simulink model "pv_mppt_inverter"  (R2014a)
settings: Solver=ode23tb  StartTime=0.0  StopTime=1  RelTol=1e-3
PreLoadFcn:
  | load('DCDCBuck_Variants');
  | load('DCACInverter_Variants');
  | load('MPPT_Variants');
  | BuckMode = 1;
  | InvMode = 1;
  | MPPTMode = 1;
  | Ts = 1e-6;
  | G = 1000;
  | PVCellIsc = 7;
  | PVCellVoc = 0.64;
  | PVCellRs = 0.001;
  | tau = 1e-4;
undefined symbols (not defined in the file or in its folder): D1, Delta, dfilt, sigbuilder_block
libraries: powerlib x48, powerlib_meascontrol x8, dsparch4 x3, simulink_extras x3, simulink x2
settings Model: Creator=cosorio  LastModifiedBy=cosorio
settings DataIOCC: LimitDataPoints=off  SignalLoggingSaveFormat=ModelDataLogs  SaveOutput=off  SignalLogging=off  DSMLogging=off  SaveTime=off  OutputTimes=[0]
settings OptimizationCC: ExpressionDepthLimit=2147483647
settings DebuggingCC: UnderspecifiedInitializationDetection=Classic  FcnCallInpInsideContextMsg=UseLocalSettings  StateNameClashWarn=warning
settings GRTTargetCC: CombineOutputUpdateFcns=off  GRTInterface=on

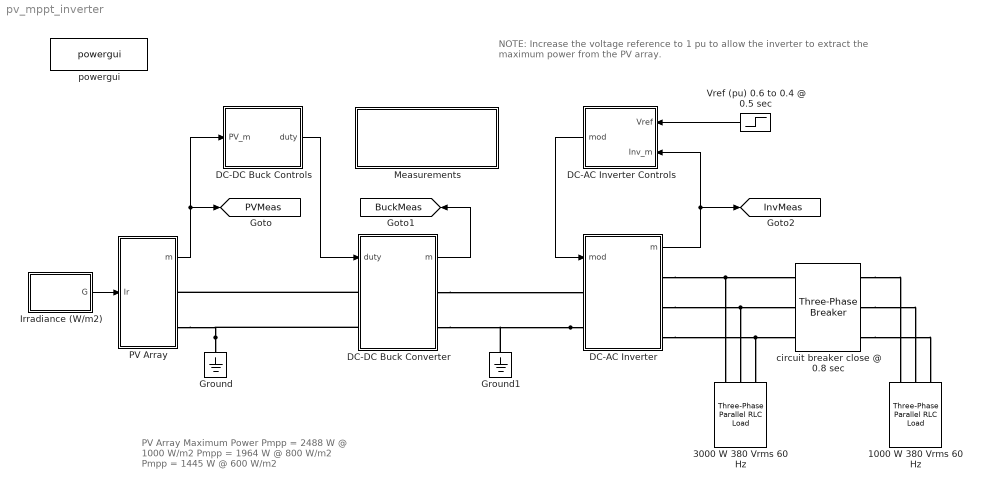
== system pv_mppt_inverter ==
  note: PV Array Maximum Power
      | Pmpp = 2488 W @ 1000 W/m2
      | Pmpp = 1964 W @ 800 W/m2
      | Pmpp = 1445 W @ 600 W/m2
  note: NOTE: Increase the voltage reference to 1 pu to allow the
      | inverter to extract the maximum power from the PV array.
  1000 W 380 Vrms 60 Hz : powerlib/Elements/Three-Phase Parallel RLC Load  LConnTagsString=A|B|C  Configuration=Y (grounded)  NominalVoltage=380  NominalFrequency=60  ActivePower=1000  InductivePower=0  CapacitivePower=0  Measurements=None  LoadType=constant Z
  3000 W 380 Vrms 60 Hz : powerlib/Elements/Three-Phase Parallel RLC Load  LConnTagsString=A|B|C  Configuration=Y (grounded)  NominalVoltage=380  NominalFrequency=60  ActivePower=3000  InductivePower=0  CapacitivePower=0  Measurements=None  LoadType=constant Z
  DC-AC Inverter : Subsystem  Variant=on
  DC-AC Inverter Controls : Subsystem  TreatAsAtomicUnit=on  SystemSampleTime=1e-4
  DC-DC Buck Controls : Subsystem  TreatAsAtomicUnit=on  SystemSampleTime=1e-4
  DC-DC Buck Converter : Subsystem  Variant=on
  Ground : powerlib/Elements/Ground  LConnTagsString=a
  Ground1 : powerlib/Elements/Ground  LConnTagsString=a
  Irradiance (W/m2) : Subsystem  Tag=STV Subsys  LoadFcn=sigbuilder_block('load');  StartFcn=sigbuilder_block('start');  StopFcn=sigbuilder_block('stop');  ClipboardFcn=sigbuilder_block('clipboard');  mask(Sigbuilder block){}
      mask help: Sigbuilder GUI
      mask init:
      | if ~strcmp(get_param(bdroot(gcbh),'SimulationStatus'),'stopped') tuvar = sigbuilder_block('maskInit'); end
      settings: CopyFcn=sigbuilder_block('copy');  DeleteFcn=sigbuilder_block('delete');  ModelCloseFcn=sigbuilder_block('modelClose');  PreSaveFcn=sigbuilder_block('preSave');  PauseFcn=sigbuilder_block('pause')  ContinueFcn=sigbuilder_block('continue')  NameChangeFcn=sigbuilder_block('namechange');  OpenFcn=sigbuilder_block('open',[124.138 6.82759 550.552 382.345 ]);  CloseFcn=sigbuilder_block('close');
      mask Display: plot(0,0,100,100,[10,10,40,40,10],[80,20,20,80,80],[40,10],[50,50], [40,27,10],[65,72,56],[40,25,25,10],[28,28,43,43]);
  Measurements : Subsystem
      mask Display: disp('System\nMeasurements');
  PV Array : Subsystem
  Vref (pu) 0.6 to 0.4 @ 0.5 sec : Step  Time=0.5  Before=0.6  After=0.4  SampleTime=1e-4
  circuit breaker close @ 0.8 sec : powerlib/Elements/Three-Phase Breaker  InitialState=open  SwitchA=on  SwitchB=on  SwitchC=on  SwitchTimes=[0.8]  External=off  BreakerResistance=0.001  SnubberResistance=1e6  SnubberCapacitance=inf  Measurements=None
  powergui : powerlib/powergui  Priority=1  SimulationMode=Continuous  SolverType=Tustin  SampleTime=Ts  frequency=60  SPID=off  DisableSnubberDevices=off  DisableRonSwitches=off  DisableVfSwitches=off  SwTol=0  Interpol=off  DisplayEquations=off  Ts=0  methode=off  frequencyindice=0  Pbase=100e6  ErrMax=1e-4  Iterations=50  UnitsV=kV  UnitsW=MW  FunctionMessages=off  echomessages=off  HookPort=off  EnableUseOfTLC=off  x0status=blocks  RestoreLinks=warning  ResistiveCurrentMeasurement=off  Frange=[0:2:500]  Ylog=off  Xlog=on  ShowGrid=off  save=off  variable=ZData  structure=InverterData  ZoomFFT=off  StartTime=0.1  cycles=3  DisplayStyle=1  fundamental=60  FreqAxis=on  MaxFrequency=24000  frequencyindicesteady=1  RmsSteady=1  display=off
  tag scope: BuckMeas=global, InvMeas=global, PVMeas=global
  wires:
  Irradiance (W/m2)/1(G) -> PV Array/1(Ir)
  DC-DC Buck Controls/1(duty) -> DC-DC Buck Converter/1(duty)
  PV Array/1(m) -> DC-DC Buck Controls/1(PV_m), [PVMeas]
  DC-DC Buck Converter/1(m) -> [BuckMeas]
  DC-AC Inverter/1(m) -> DC-AC Inverter Controls/2(Inv_m), [InvMeas]
  DC-AC Inverter Controls/1(mod) -> DC-AC Inverter/1(mod)
  Vref (pu) 0.6 to 0.4 @ 0.5 sec/1 -> DC-AC Inverter Controls/1(Vref)
  connections:
  Ground/LConn1 -- DC-DC Buck Converter/LConn2 -- PV Array/RConn2
  DC-DC Buck Converter/LConn1 -- PV Array/RConn1
  DC-DC Buck Converter/RConn1 -- DC-AC Inverter/LConn1
  DC-AC Inverter/LConn2 -- DC-DC Buck Converter/RConn2 -- Ground1/LConn1
  DC-AC Inverter/RConn1 -- circuit breaker close @ 0.8 sec/LConn1 -- 3000 W 380 Vrms 60 Hz/LConn1
  DC-AC Inverter/RConn2 -- 3000 W 380 Vrms 60 Hz/LConn2 -- circuit breaker close @ 0.8 sec/LConn2
  DC-AC Inverter/RConn3 -- circuit breaker close @ 0.8 sec/LConn3 -- 3000 W 380 Vrms 60 Hz/LConn3
  circuit breaker close @ 0.8 sec/RConn3 -- 1000 W 380 Vrms 60 Hz/LConn3
  circuit breaker close @ 0.8 sec/RConn2 -- 1000 W 380 Vrms 60 Hz/LConn2
  circuit breaker close @ 0.8 sec/RConn1 -- 1000 W 380 Vrms 60 Hz/LConn1

== system pv_mppt_inverter/DC-AC Inverter ==
  mod : Inport
  AVG Voltage : Subsystem  VariantControl=DCACInverterAVG
  Detailed : Subsystem  VariantControl=DCACInverterDET
  in + : PMIOPort  Port=1  Side=Left
  in -- : PMIOPort  Port=2  Side=Left
  A : PMIOPort  Port=3  Side=Right
  B : PMIOPort  Port=4  Side=Right
  C : PMIOPort  Port=5  Side=Right
  m : Outport

== system pv_mppt_inverter/DC-AC Inverter Controls ==
  note: NOTE: Regulating the inverter to a desired setpoint voltage for
      | a fixed load will limit the current flowing through the inverter.
      | As can be seen from the simulation, this results in the PV array
      | NOT necessarily operating at peak efficiency.
  Vref : Inport  SampleTime=1e-4
  Inv_m : Inport  Port=2  SampleTime=1e-4
  Bus Selector3 : BusSelector  OutputSignals=VabcInv
  Voltage Regulator : Subsystem
  mod : Outport
  wires:
  Bus Selector3/1 -> Voltage Regulator/2(Vabc (pu))  "<VabcInv>"
  Inv_m/1 -> Bus Selector3/1
  Vref/1 -> Voltage Regulator/1(Vd_ref (pu))
  Voltage Regulator/1(Vabc_inv) -> mod/1

== system pv_mppt_inverter/DC-DC Buck Controls ==
  PV_m : Inport  SampleTime=1e-4
  Bus Selector : BusSelector  OutputSignals=PVVocREF (V),PVVoltage (V),PVCurrent (A)
  MPPT Algorithm : ModelReference  ModelNameDialog=FractionalOCVoltage.slx  Variant=on  ModelReferenceVersion=1.167  CopyOfModelName=FractionalOCVoltage.slx  DefaultDataLogging=on
  Signal Conditioning : Subsystem
  duty : Outport
  wires:
  PV_m/1 -> Bus Selector/1
  Bus Selector/2 -> Signal Conditioning/2(In2)  "<PVVoltage (V)>"
  Bus Selector/1 -> Signal Conditioning/1(In1)  "<PVVocREF (V)>"
  MPPT Algorithm/1 -> duty/1
  Signal Conditioning/1(Out1) -> MPPT Algorithm/1
  Signal Conditioning/2(Out2) -> MPPT Algorithm/2
  Bus Selector/3 -> Signal Conditioning/3(In3)  "<PVCurrent (A)>"
  Signal Conditioning/3(Out3) -> MPPT Algorithm/3

== system pv_mppt_inverter/DC-DC Buck Converter ==
  duty : Inport
  AVG Voltage : Subsystem  VariantControl=DCDCBuckAVG
  Detailed : Subsystem  VariantControl=DCDCBuckDET
  Low Level : Subsystem  VariantControl=DCDCBuckLOW
  in + : PMIOPort  Port=1  Side=Left
  in -- : PMIOPort  Port=2  Side=Left
  out + : PMIOPort  Port=3  Side=Right
  out -- : PMIOPort  Port=4  Side=Right
  m : Outport

== system pv_mppt_inverter/Irradiance (W//m2) ==
  Demux : Demux  Tag=STV Demux  Outputs=1
  FromWs : FromWorkspace  Tag=STV FromWs  VariableName=tuvar  SampleTime=0
      SigBuilderData=|
      | common.afterFinalStr = 'Extrapolate'
      | common.sampleTime = '0'
      | dataSet(1).timeRange = [0 1]
      | dataSet(1).name = 'Constant Irradiance'
      | dataSet(2).timeRange = [0 1]
      | dataSet(2).name = 'Step Irradiance'
      | dataSet(3).timeRange = [0 1]
      | dataSet(3).name = 'Trapezoidal Irradiance'
      | sbobj.Groups(1).Name = 'Constant Irradiance'
      | sbobj.Groups(1).Signals.Name = 'G'
      | sbobj.Groups(1).Signals.XData = [0 1]
      | sbobj.Groups(1).Signals.YData = [800 800]
      | sbobj.Groups(1).TimeRange = [0 1]
      | sbobj.Groups(2).Name = 'Step Irradiance'
      | sbobj.Groups(2).Signals.Name = 'G'
      | sbobj.Groups(2).Signals.XData = [0 0.5 0.5 1]
      | sbobj.Groups(2).Signals.YData = [600 600 1000 1000]
      | sbobj.Groups(2).TimeRange = [0 1]
      | sbobj.Groups(3).Name = 'Trapezoidal Irradiance'
      | sbobj.Groups(3).Signals.Name = 'G'
      | sbobj.Groups(3).Signals.XData = [0 0.2 0.3 0.5 0.7 0.9 1]
      | sbobj.Groups(3).Signals.YData = [800 800 600 600 1000 1000 800]
      | sbobj.Groups(3).TimeRange = [0 1]
  G : Outport  Tag=STV Outport
  wires:
  Demux/1 -> G/1
  FromWs/1 -> Demux/1

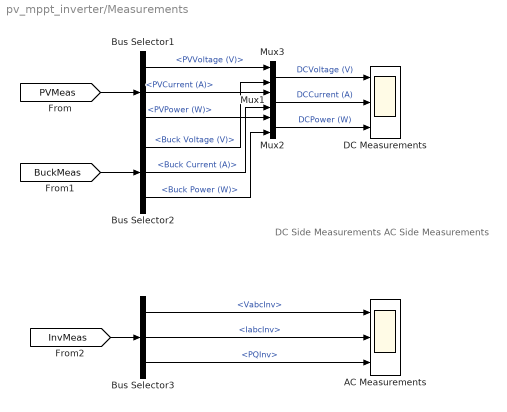
== system pv_mppt_inverter/Measurements ==
  note: DC Side Measurements
      |
      |
      |
      |
      |
      |
      |
      |
      |
      |
      | AC Side Measurements
  AC Measurements : Scope  NumInputPorts=3
      settings: YMin=-2~-1~-0.5  YMax=2~1~1  SaveName=InverterData
  Bus Selector1 : BusSelector  OutputSignals=PVVoltage (V),PVCurrent (A),PVPower (W)
  Bus Selector2 : BusSelector  OutputSignals=Buck Voltage (V),Buck Current (A),Buck Power (W)
  Bus Selector3 : BusSelector  OutputSignals=VabcInv,IabcInv,PQInv
  DC Measurements : Scope  NumInputPorts=3
      settings: YMin=0~0~0  YMax=250~40~3000  SaveName=PVArrayData
  Mux1 : Mux  Inputs=2
  Mux2 : Mux  Inputs=2
  Mux3 : Mux  Inputs=2
  wires:
  Bus Selector1/1 -> Mux3/1  "<PVVoltage (V)>"
  Bus Selector1/2 -> Mux1/1  "<PVCurrent (A)>"
  Bus Selector1/3 -> Mux2/1  "<PVPower (W)>"
  Bus Selector2/1 -> Mux3/2  "<Buck Voltage (V)>"
  Bus Selector2/2 -> Mux1/2  "<Buck Current (A)>"
  Bus Selector2/3 -> Mux2/2  "<Buck Power (W)>"
  Mux3/1 -> DC Measurements/1  "DCVoltage (V)"
  Mux1/1 -> DC Measurements/2  "DCCurrent (A)"
  Mux2/1 -> DC Measurements/3  "DCPower (W)"
  [PVMeas] -> Bus Selector1/1
  [BuckMeas] -> Bus Selector2/1
  [InvMeas] -> Bus Selector3/1
  Bus Selector3/1 -> AC Measurements/1  "<VabcInv>"
  Bus Selector3/2 -> AC Measurements/2  "<IabcInv>"
  Bus Selector3/3 -> AC Measurements/3  "<PQInv>"

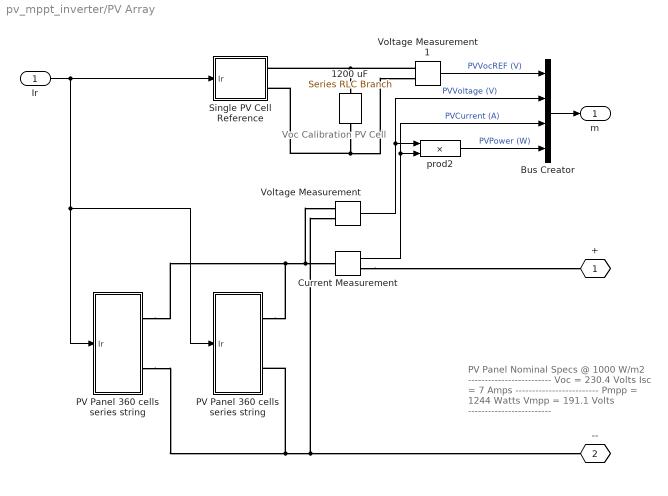
== system pv_mppt_inverter/PV Array ==
  note: Voc Calibration PV Cell
  note: PV Panel
      | Nominal Specs @ 1000 W/m2
      | -------------------------
      | Voc = 230.4 Volts
      | Isc = 7 Amps
      | -------------------------
      | Pmpp = 1244 Watts
      | Vmpp = 191.1 Volts
      | -------------------------
  Ir : Inport
  1200 uF : powerlib/Elements/Series RLC Branch  LConnTagsString=__new0  RConnTagsString=__new0  BranchType=C  Resistance=0.05  Inductance=1e-3  SetiL0=off  InitialCurrent=0  Capacitance=1200e-6  Setx0=on  InitialVoltage=PVCellVoc  Measurements=None
  Bus Creator : BusCreator
  Current Measurement : powerlib/Measurements/Current Measurement  PhasorSimulation=off  OutputType=Complex  PSBequivalent=0
  PV Panel 360 cells series string : Subsystem  mask(Solar Cell){Isc=PVCellIsc, Voc=PVCellVoc*360, Ir0=1000, N=1.5*360, Rs=PVCellRs*360, Rp=1000*360, tau=tau}
      mask prompts: Isc "Short-circuit current, Isc (A):"; Voc "Open-circuit voltage, Voc (V):"; Ir0 "Irradiance used for measurements, Ir0 (W/m2):"; N "Quality factor, N:"; Rs "Series resistance, Rs (ohms):"; Rp "Parallel resistance, Rp (ohms):"; tau "Time constant (sec):"
      mask help:
      | Simulink implementation of an idividual solar cell. The cell is modelled as a parallel combination of a current source, an exponential diode and an internal resistance Rp, connected in series with a resistance Rs.
      | The cell output current is given by:
      |
      | Ipv = Iph - Is * (exp((V + I*Rs)/(N*Vt)) - 1) - (V + I*Rs)/Rp
      |
      | Where Iph is the solar generated current, Is is the diode saturation current, Vt is the thermal voltage, N is the diode quality factor (emission coefficient).
      |
      | A first order transfer function is used to break the algebraic loop. The time constant of this transfer function should be adjusted such that it will not significantly affect your model dynamics.
      mask init:
      | %% Cell thermal voltage calculation
      | T = 25 + 273;   % Device operating temperature (oC)
      | k = 1.3806e-23; % Boltzman constant (J/oK)
      | q = 1.602e-19;  % Elementary charge on an electron (oC)
      | Vt = k*T/q;     % Thermal voltage
      | 
      | %% Diode saturation current calculation
      | Is = Isc/(exp(Voc/(N*Vt))-1);
  "PV Panel 360 cells series string " : Subsystem  mask(Solar Cell){Isc=PVCellIsc, Voc=PVCellVoc*360, Ir0=1000, N=1.5*360, Rs=PVCellRs*360, Rp=1000*360, tau=tau}
      mask prompts: Isc "Short-circuit current, Isc (A):"; Voc "Open-circuit voltage, Voc (V):"; Ir0 "Irradiance used for measurements, Ir0 (W/m2):"; N "Quality factor, N:"; Rs "Series resistance, Rs (ohms):"; Rp "Parallel resistance, Rp (ohms):"; tau "Time constant (sec):"
      mask help:
      | Simulink implementation of an idividual solar cell. The cell is modelled as a parallel combination of a current source, an exponential diode and an internal resistance Rp, connected in series with a resistance Rs.
      | The cell output current is given by:
      |
      | Ipv = Iph - Is * (exp((V + I*Rs)/(N*Vt)) - 1) - (V + I*Rs)/Rp
      |
      | Where Iph is the solar generated current, Is is the diode saturation current, Vt is the thermal voltage, N is the diode quality factor (emission coefficient).
      |
      | A first order transfer function is used to break the algebraic loop. The time constant of this transfer function should be adjusted such that it will not significantly affect your model dynamics.
      mask init: same as pv_mppt_inverter/PV Array/PV Panel 360 cells series string
  Single PV Cell Reference : Subsystem  mask(Solar Cell){Isc=PVCellIsc, Voc=PVCellVoc, Ir0=1000, N=1.5, Rs=PVCellRs, Rp=1000, tau=tau}
      mask prompts: Isc "Short-circuit current, Isc (A):"; Voc "Open-circuit voltage, Voc (V):"; Ir0 "Irradiance used for measurements, Ir0 (W/m2):"; N "Quality factor, N:"; Rs "Series resistance, Rs (ohms):"; Rp "Parallel resistance, Rp (ohms):"; tau "Time constant (sec):"
      mask help:
      | Simulink implementation of an idividual solar cell. The cell is modelled as a parallel combination of a current source, an exponential diode and an internal resistance Rp, connected in series with a resistance Rs.
      | The cell output current is given by:
      |
      | Ipv = Iph - Is * (exp((V + I*Rs)/(N*Vt)) - 1) - (V + I*Rs)/Rp
      |
      | Where Iph is the solar generated current, Is is the diode saturation current, Vt is the thermal voltage, N is the diode quality factor (emission coefficient).
      |
      | A first order transfer function is used to break the algebraic loop. The time constant of this transfer function should be adjusted such that it will not significantly affect your model dynamics.
      mask init: same as pv_mppt_inverter/PV Array/PV Panel 360 cells series string
  Voltage Measurement : powerlib/Measurements/Voltage Measurement  PhasorSimulation=off  OutputType=Complex  PSBequivalent=0
  Voltage Measurement1 : powerlib/Measurements/Voltage Measurement  PhasorSimulation=off  OutputType=Complex  PSBequivalent=0
  prod2 : Product  Inputs=**
  + : PMIOPort  Tag=PMCPort  Port=1  Side=Right
  -- : PMIOPort  Tag=PMCPort  Port=2  Side=Right
  m : Outport
  wires:
  prod2/1 -> Bus Creator/4  "PVPower (W)"
  Current Measurement/1 -> prod2/2, Bus Creator/3  "PVCurrent (A)"
  Voltage Measurement1/1 -> Bus Creator/1  "PVVocREF (V)"
  Ir/1 -> PV Panel 360 cells series string/1(Ir), "PV Panel 360 cells series string "/1(Ir), Single PV Cell Reference/1(Ir)
  Bus Creator/1 -> m/1
  Voltage Measurement/1 -> prod2/1, Bus Creator/2  "PVVoltage (V)"
  connections:
  Single PV Cell Reference/RConn1 -- 1200 uF/LConn1 -- Voltage Measurement1/LConn1
  Single PV Cell Reference/RConn2 -- Voltage Measurement1/LConn2 -- 1200 uF/RConn1
  "PV Panel 360 cells series string "/RConn2 -- --/RConn1 -- Voltage Measurement/LConn2 -- PV Panel 360 cells series string/RConn2
  Current Measurement/RConn1 -- +/RConn1
  "PV Panel 360 cells series string "/RConn1 -- Current Measurement/LConn1 -- Voltage Measurement/LConn1 -- PV Panel 360 cells series string/RConn1

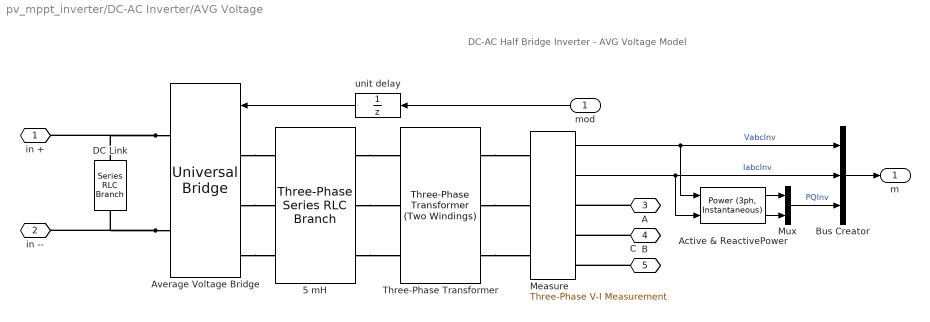
== system pv_mppt_inverter/DC-AC Inverter/AVG Voltage ==
  note: DC-AC Half Bridge Inverter - AVG Voltage Model
  mod : Inport
  "5 mH " : powerlib/Elements/Three-Phase Series RLC Branch  LConnTagsString=A|B|C  RConnTagsString=A|B|C  BranchType=RL  Resistance=0.25  Inductance=5e-3  Capacitance=1.0  Measurements=None
  Active & ReactivePower : powerlib_meascontrol/Measurements/Power (3ph, Instantaneous)
  Average Voltage Bridge : powerlib/Power Electronics/Universal Bridge  Arms=3  SnubberResistance=1e5  SnubberCapacitance=inf  Device=Average-model based VSC  Ron=1e-4  Lon=0  ForwardVoltages="[  0  0  ]"  ForwardVoltage=0  GTOparameters=[ 10e-6 , 20e-6 ]  IGBTparameters=[ 1e-6 , 2e-6 ]  Measurements=None  Measurements_2=None  converterType=Rectifier
  Bus Creator : BusCreator  Inputs=3
  DC Link : powerlib/Elements/Series RLC Branch  LConnTagsString=__new0  RConnTagsString=__new0  BranchType=RC  Resistance=0.25  Inductance=30e-6  SetiL0=off  InitialCurrent=0  Capacitance=1200e-6  Setx0=on  InitialVoltage=128.5  Measurements=None
  Measure : powerlib/Measurements/Three-Phase V-I Measurement  VoltageMeasurement=phase-to-ground  SetLabelV=off  LabelV=V1  Vpu=on  VpuLL=off  CurrentMeasurement=yes  SetLabelI=off  LabelI=I1  Ipu=on  Pbase=3000*sqrt(3)  Vbase=380  OutputType=Magnitude  PhasorSimulation=off  PSBequivalent=0
  Mux : Mux  Inputs=2
  Three-Phase Transformer : powerlib/Elements/Three-Phase Transformer (Two Windings)  Winding1Connection=Delta (D1)  UNITS=pu  NominalPower=[3000*sqrt(3), 60 ]  Winding1=[110 0.002 0.08]  Winding2Connection=Yg  Winding2=[380 0.002 0.079998]  SetSaturation=off  Rm=500  Lm=500  Saturation=[0 0;0.0024 1.2;1 1.52]  Hysteresis=off  DataFile='hysteresis'  SetInitialFlux=off  InitialFluxes=[0.8 -0.8 0.69998]  Measurements=None  MoreParameters=off  BreakLoop=off  DataType=off  TransfoNumber=1
  unit delay : UnitDelay  SampleTime=1e-4
  in + : PMIOPort  Port=1  Side=Left
  in -- : PMIOPort  Port=2  Side=Left
  A : PMIOPort  Port=3  Side=Right
  B : PMIOPort  Port=4  Side=Right
  C : PMIOPort  Port=5  Side=Right
  m : Outport
  wires:
  Mux/1 -> Bus Creator/3  "PQInv"
  Bus Creator/1 -> m/1
  Measure/2 -> Active & ReactivePower/2, Bus Creator/2  "IabcInv"
  Measure/1 -> Active & ReactivePower/1, Bus Creator/1  "VabcInv"
  mod/1 -> unit delay/1
  unit delay/1 -> Average Voltage Bridge/1
  Active & ReactivePower/1 -> Mux/1
  Active & ReactivePower/2 -> Mux/2
  connections:
  C/RConn1 -- Measure/RConn3
  B/RConn1 -- Measure/RConn2
  A/RConn1 -- Measure/RConn1
  Average Voltage Bridge/LConn3 -- "5 mH "/LConn3
  Average Voltage Bridge/LConn2 -- "5 mH "/LConn2
  Average Voltage Bridge/LConn1 -- "5 mH "/LConn1
  Average Voltage Bridge/RConn2 -- DC Link/RConn1 -- in --/RConn1
  Average Voltage Bridge/RConn1 -- DC Link/LConn1 -- in +/RConn1
  "5 mH "/RConn1 -- Three-Phase Transformer/LConn1
  Three-Phase Transformer/RConn1 -- Measure/LConn1
  "5 mH "/RConn2 -- Three-Phase Transformer/LConn2
  Three-Phase Transformer/RConn2 -- Measure/LConn2
  "5 mH "/RConn3 -- Three-Phase Transformer/LConn3
  Three-Phase Transformer/RConn3 -- Measure/LConn3

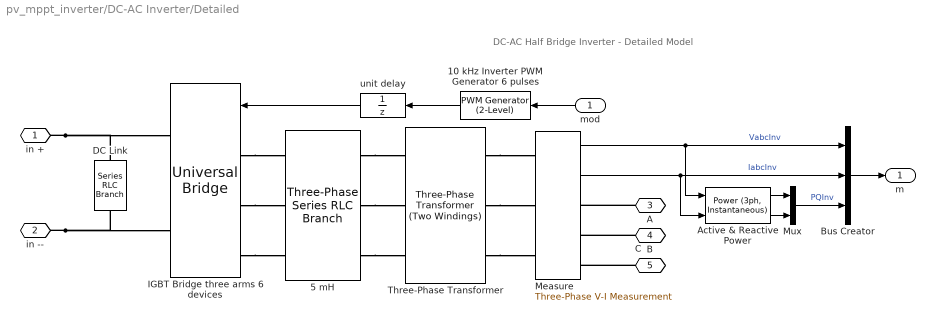
== system pv_mppt_inverter/DC-AC Inverter/Detailed ==
  note: DC-AC Half Bridge Inverter - Detailed Model
  mod : Inport
  10 kHz Inverter PWM Generator 6 pulses : powerlib_meascontrol/Pulse & Signal Generators/PWM Generator (2-Level)  ModulatorType=Three-phase bridge (6 pulses)  ModulatorMode=Unsynchronized  nF=27  Fc=1e04  ModulatingSignals=off  m=0.8  Freq=60  Phase=0  Ts=Ts
  "5 mH " : powerlib/Elements/Three-Phase Series RLC Branch  LConnTagsString=A|B|C  RConnTagsString=A|B|C  BranchType=RL  Resistance=0.25  Inductance=5e-3  Capacitance=1.0  Measurements=None
  Active & Reactive Power : powerlib_meascontrol/Measurements/Power (3ph, Instantaneous)
  Bus Creator : BusCreator  Inputs=3
  DC Link : powerlib/Elements/Series RLC Branch  LConnTagsString=__new0  RConnTagsString=__new0  BranchType=RC  Resistance=0.25  Inductance=30e-6  SetiL0=off  InitialCurrent=0  Capacitance=1200e-6  Setx0=on  InitialVoltage=180  Measurements=None
  IGBT Bridge three arms 6 devices : powerlib/Power Electronics/Universal Bridge  Arms=3  SnubberResistance=1e5  SnubberCapacitance=inf  Device=IGBT / Diodes  Ron=1e-4  Lon=0  ForwardVoltages="[  0  0  ]"  ForwardVoltage=0  GTOparameters=[ 10e-6 , 20e-6 ]  IGBTparameters=[ 1e-6 , 2e-6 ]  Measurements=None  Measurements_2=None  converterType=Rectifier
  Measure : powerlib/Measurements/Three-Phase V-I Measurement  VoltageMeasurement=phase-to-ground  SetLabelV=off  LabelV=V1  Vpu=on  VpuLL=off  CurrentMeasurement=yes  SetLabelI=off  LabelI=I1  Ipu=on  Pbase=3000*sqrt(3)  Vbase=380  OutputType=Magnitude  PhasorSimulation=off  PSBequivalent=0
  Mux : Mux  Inputs=2
  Three-Phase Transformer : powerlib/Elements/Three-Phase Transformer (Two Windings)  Winding1Connection=Delta (D1)  UNITS=pu  NominalPower=[3000*sqrt(3) , 60 ]  Winding1=[110, 0.002 , 0.08 ]  Winding2Connection=Yg  Winding2=[380 , 0.002 , 0.08 ]  SetSaturation=off  Rm=500  Lm=500  Saturation=[ 0,0 ; 0.0024,1.2 ; 1.0,1.52 ]  Hysteresis=off  DataFile='hysteresis'  SetInitialFlux=off  InitialFluxes=[ 0.8 , -0.8 , 0.7 ]  Measurements=None  MoreParameters=off  BreakLoop=off  DataType=off  TransfoNumber=1
  unit delay : UnitDelay  SampleTime=Ts
  in + : PMIOPort  Port=1  Side=Left
  in -- : PMIOPort  Port=2  Side=Left
  A : PMIOPort  Port=3  Side=Right
  B : PMIOPort  Port=4  Side=Right
  C : PMIOPort  Port=5  Side=Right
  m : Outport
  wires:
  10 kHz Inverter PWM Generator 6 pulses/1 -> unit delay/1
  mod/1 -> 10 kHz Inverter PWM Generator 6 pulses/1
  Measure/1 -> Active & Reactive Power/1, Bus Creator/1  "VabcInv"
  Measure/2 -> Active & Reactive Power/2, Bus Creator/2  "IabcInv"
  Bus Creator/1 -> m/1
  unit delay/1 -> IGBT Bridge three arms 6 devices/1
  Mux/1 -> Bus Creator/3  "PQInv"
  Active & Reactive Power/1 -> Mux/1
  Active & Reactive Power/2 -> Mux/2
  connections:
  in +/RConn1 -- DC Link/LConn1 -- IGBT Bridge three arms 6 devices/RConn1
  in --/RConn1 -- DC Link/RConn1 -- IGBT Bridge three arms 6 devices/RConn2
  IGBT Bridge three arms 6 devices/LConn1 -- "5 mH "/LConn1
  IGBT Bridge three arms 6 devices/LConn2 -- "5 mH "/LConn2
  IGBT Bridge three arms 6 devices/LConn3 -- "5 mH "/LConn3
  A/RConn1 -- Measure/RConn1
  B/RConn1 -- Measure/RConn2
  C/RConn1 -- Measure/RConn3
  "5 mH "/RConn1 -- Three-Phase Transformer/LConn1
  "5 mH "/RConn2 -- Three-Phase Transformer/LConn2
  "5 mH "/RConn3 -- Three-Phase Transformer/LConn3
  Three-Phase Transformer/RConn3 -- Measure/LConn3
  Three-Phase Transformer/RConn2 -- Measure/LConn2
  Three-Phase Transformer/RConn1 -- Measure/LConn1

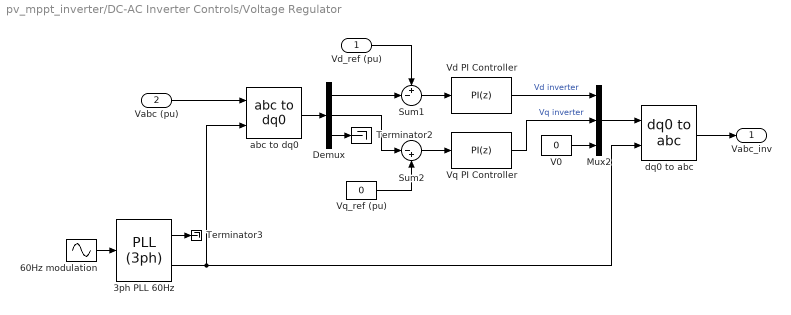
== system pv_mppt_inverter/DC-AC Inverter Controls/Voltage Regulator ==
  Vd_ref (pu) : Inport
  Vabc (pu) : Inport  Port=2
  " 3ph PLL 60Hz" : powerlib_meascontrol/PLL/PLL (3ph)  Fmin=45  Par_Init=[0, 60]  ParK=[180, 3200, 1]  TcD=1e-4  MaxRateChangeFreq=12  FilterCutOffFreq=25  Ts=1e-4  AGC=off
  60Hz modulation : Sin  Frequency=2*pi*60  Phase=[-2*pi/3, 0, 2*pi/3]  SampleTime=1e-4
  Demux : Demux  Outputs=3
  Mux2 : Mux  Inputs=3
  Sum1 : Sum  Inputs=+-|  SaturateOnIntegerOverflow=on  InputSameDT=on  OutDataTypeStr=Inherit: Same as first input
  Sum2 : Sum  Inputs=|-+  SaturateOnIntegerOverflow=on  InputSameDT=on  OutDataTypeStr=Inherit: Same as first input
  Terminator2 : Terminator
  Terminator3 : Terminator
  V0 : Constant  Value=0
  Vd PI Controller : simulink/Continuous/PID Controller  Controller=PI  TimeDomain=Discrete-time  SampleTime=1e-4  IntegratorMethod=Forward Euler  FilterMethod=Forward Euler  Form=Parallel  P=1.08675469995769  I=2143.9241567618  D=0  N=100  InitialConditionSource=internal  InitialConditionForIntegrator=0  InitialConditionForFilter=0  ExternalReset=none  LimitOutput=on  UpperSaturationLimit=1  LowerSaturationLimit=0  LinearizeAsGain=on  AntiWindupMode=clamping  Kb=1  TrackingMode=off  Kt=1  PParamMin=[]  PParamMax=[]  IParamMin=[]  IParamMax=[]  DParamMin=[]  DParamMax=[]  NParamMin=[]  NParamMax=[]  KbParamMin=[]  KbParamMax=[]  KtParamMin=[]  KtParamMax=[]  POutMin=[]  POutMax=[]  IOutMin=[]  IOutMax=[]  DOutMin=[]  DOutMax=[]  NOutMin=[]  NOutMax=[]  KbOutMin=[]  KbOutMax=[]  KtOutMin=[]  KtOutMax=[]  IntegratorOutMin=[]  IntegratorOutMax=[]  FilterOutMin=[]  FilterOutMax=[]  SumOutMin=[]  SumOutMax=[]  SumI1OutMin=[]  SumI1OutMax=[]  SumI2OutMin=[]  SumI2OutMax=[]  SumI3OutMin=[]  SumI3OutMax=[]  SumDOutMin=[]  SumDOutMax=[]  SaturationOutMin=[]  SaturationOutMax=[]  IntegratorContinuousStateAttributes=''  IntegratorStateMustResolveToSignalObject=off  IntegratorRTWStateStorageClass=Auto  FilterContinuousStateAttributes=''  FilterStateMustResolveToSignalObject=off  FilterRTWStateStorageClass=Auto
  Vq PI Controller : simulink/Continuous/PID Controller  Controller=PI  TimeDomain=Discrete-time  SampleTime=1e-4  IntegratorMethod=Forward Euler  FilterMethod=Forward Euler  Form=Parallel  P=1.08675469995769  I=2143.9241567618  D=0  N=100  InitialConditionSource=internal  InitialConditionForIntegrator=0  InitialConditionForFilter=0  ExternalReset=none  LimitOutput=on  UpperSaturationLimit=1  LowerSaturationLimit=-1  LinearizeAsGain=on  AntiWindupMode=clamping  Kb=1  TrackingMode=off  Kt=1  PParamMin=[]  PParamMax=[]  IParamMin=[]  IParamMax=[]  DParamMin=[]  DParamMax=[]  NParamMin=[]  NParamMax=[]  KbParamMin=[]  KbParamMax=[]  KtParamMin=[]  KtParamMax=[]  POutMin=[]  POutMax=[]  IOutMin=[]  IOutMax=[]  DOutMin=[]  DOutMax=[]  NOutMin=[]  NOutMax=[]  KbOutMin=[]  KbOutMax=[]  KtOutMin=[]  KtOutMax=[]  IntegratorOutMin=[]  IntegratorOutMax=[]  FilterOutMin=[]  FilterOutMax=[]  SumOutMin=[]  SumOutMax=[]  SumI1OutMin=[]  SumI1OutMax=[]  SumI2OutMin=[]  SumI2OutMax=[]  SumI3OutMin=[]  SumI3OutMax=[]  SumDOutMin=[]  SumDOutMax=[]  SaturationOutMin=[]  SaturationOutMax=[]  IntegratorContinuousStateAttributes=''  IntegratorStateMustResolveToSignalObject=off  IntegratorRTWStateStorageClass=Auto  FilterContinuousStateAttributes=''  FilterStateMustResolveToSignalObject=off  FilterRTWStateStorageClass=Auto
  Vq_ref (pu) : Constant  Value=0
  abc to dq0 : powerlib_meascontrol/Transformations/abc to dq0  Alignment=90 degrees behind phase A axis
  dq0 to abc : powerlib_meascontrol/Transformations/dq0 to abc  Alignment=90 degrees behind phase A axis
  Vabc_inv : Outport
  wires:
  Vd PI Controller/1 -> Mux2/1  "Vd inverter"
  " 3ph PLL 60Hz"/2 -> dq0 to abc/2, abc to dq0/2
  dq0 to abc/1 -> Vabc_inv/1
  Mux2/1 -> dq0 to abc/1
  Sum1/1 -> Vd PI Controller/1
  Vabc (pu)/1 -> abc to dq0/1
  abc to dq0/1 -> Demux/1
  Sum2/1 -> Vq PI Controller/1
  Vq_ref (pu)/1 -> Sum2/2
  Demux/2 -> Sum2/1
  Vq PI Controller/1 -> Mux2/2  "Vq inverter"
  V0/1 -> Mux2/3
  Demux/1 -> Sum1/2
  Vd_ref (pu)/1 -> Sum1/1
  Demux/3 -> Terminator2/1
  " 3ph PLL 60Hz"/1 -> Terminator3/1
  60Hz modulation/1 -> " 3ph PLL 60Hz"/1

== system pv_mppt_inverter/DC-DC Buck Controls/Signal Conditioning ==
  In1 : Inport
  In2 : Inport  Port=2
  In3 : Inport  Port=3
  lowpass filter : dsparch4/Biquad Filter  Tag=BlockMethodSubSystem  IIRFiltStruct=Direct form II  CoeffSource=Specify via dialog  BiQuadCoeffs=[1 2 1 1 -1.84752974002334 0.907455977110453;1 2 1 1 -1.70200879073573 0.757214929023218;1 2 1 1 -1.60523823546143 0.657305536461053;1 2 1 1 -1.55731859382262 0.607831579487681]  a0Flag=Warning  IC=0  ICnum=0  ICden=0  InputProcessing=Columns as channels (frame based)  denAccumFracLength=30  denProdOutputFracLength=30  secondMemoryFracLength=15  roundingMode=Floor  overflowMode=off  ScaleValues=[0.0149815592717771;0.0138015345718716;0.0130168252499061;0.0126282464162658;1]  optimizeScaleValues=on  ScaleValueMode=Specify via input port (g)  scaleValueFracLength=14  FilterSource=Specify via dialog  dfiltObjectName=dfilt.df2tsos([1 0.3 0.4],[1 0.1 0.2])
  "lowpass filter " : dsparch4/Biquad Filter  Tag=BlockMethodSubSystem  IIRFiltStruct=Direct form II  CoeffSource=Specify via dialog  BiQuadCoeffs=[1 2 1 1 -1.84752974002334 0.907455977110453;1 2 1 1 -1.70200879073573 0.757214929023218;1 2 1 1 -1.60523823546143 0.657305536461053;1 2 1 1 -1.55731859382262 0.607831579487681]  a0Flag=Warning  IC=0  ICnum=0  ICden=0  InputProcessing=Columns as channels (frame based)  denAccumFracLength=30  denProdOutputFracLength=30  secondMemoryFracLength=15  roundingMode=Floor  overflowMode=off  ScaleValues=[0.0149815592717771;0.0138015345718716;0.0130168252499061;0.0126282464162658;1]  optimizeScaleValues=on  ScaleValueMode=Specify via input port (g)  scaleValueFracLength=14  FilterSource=Specify via dialog  dfiltObjectName=dfilt.df2tsos([1 0.3 0.4],[1 0.1 0.2])
  "lowpass filter  " : dsparch4/Biquad Filter  Tag=BlockMethodSubSystem  IIRFiltStruct=Direct form II  CoeffSource=Specify via dialog  BiQuadCoeffs=[1 2 1 1 -1.84752974002334 0.907455977110453;1 2 1 1 -1.70200879073573 0.757214929023218;1 2 1 1 -1.60523823546143 0.657305536461053;1 2 1 1 -1.55731859382262 0.607831579487681]  a0Flag=Warning  IC=0  ICnum=0  ICden=0  InputProcessing=Columns as channels (frame based)  denAccumFracLength=30  denProdOutputFracLength=30  secondMemoryFracLength=15  roundingMode=Floor  overflowMode=off  ScaleValues=[0.0149815592717771;0.0138015345718716;0.0130168252499061;0.0126282464162658;1]  optimizeScaleValues=on  ScaleValueMode=Specify via input port (g)  scaleValueFracLength=14  FilterSource=Specify via dialog  dfiltObjectName=dfilt.df2tsos([1 0.3 0.4],[1 0.1 0.2])
  Out1 : Outport
  Out2 : Outport  Port=2
  Out3 : Outport  Port=3
  wires:
  In1/1 -> lowpass filter/1
  lowpass filter/1 -> Out1/1
  In2/1 -> "lowpass filter "/1
  "lowpass filter "/1 -> Out2/1
  In3/1 -> "lowpass filter  "/1
  "lowpass filter  "/1 -> Out3/1

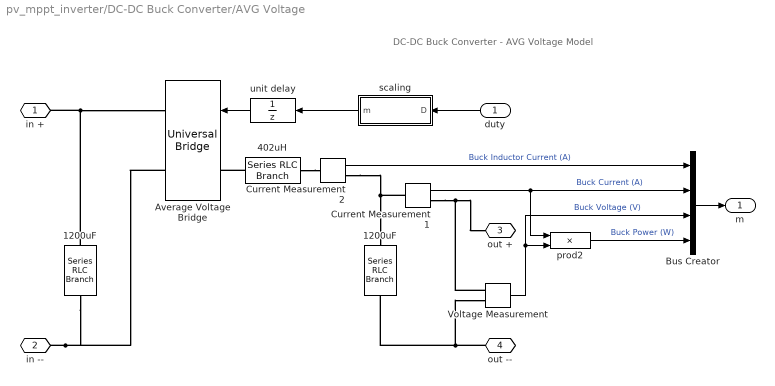
== system pv_mppt_inverter/DC-DC Buck Converter/AVG Voltage ==
  note: DC-DC Buck Converter - AVG Voltage Model
  duty : Inport
  1200uF : powerlib/Elements/Series RLC Branch  LConnTagsString=__new0  RConnTagsString=__new0  BranchType=RC  Resistance=0.25  Inductance=30e-6  SetiL0=off  InitialCurrent=0  Capacitance=1200e-6  Setx0=on  InitialVoltage=128.5  Measurements=None
  "1200uF " : powerlib/Elements/Series RLC Branch  LConnTagsString=__new0  RConnTagsString=__new0  BranchType=RC  Resistance=0.25  Inductance=30e-6  SetiL0=off  InitialCurrent=0  Capacitance=1200e-6  Setx0=on  InitialVoltage=186.4  Measurements=None
  402uH : powerlib/Elements/Series RLC Branch  LConnTagsString=__new0  RConnTagsString=__new0  BranchType=RL  Resistance=0.1  Inductance=402e-6  SetiL0=off  InitialCurrent=18  Capacitance=1e-6  Setx0=off  InitialVoltage=0  Measurements=None
  Average Voltage Bridge : powerlib/Power Electronics/Universal Bridge  Arms=1  SnubberResistance=1e5  SnubberCapacitance=inf  Device=Average-model based VSC  Ron=1e-4  Lon=0  ForwardVoltages="[  0  0  ]"  ForwardVoltage=0  GTOparameters=[ 10e-6 , 20e-6 ]  IGBTparameters=[ 1e-6 , 2e-6 ]  Measurements=None  Measurements_2=None  converterType=Rectifier
  Bus Creator : BusCreator
  Current Measurement1 : powerlib/Measurements/Current Measurement  PhasorSimulation=off  OutputType=Complex  PSBequivalent=0
  Current Measurement2 : powerlib/Measurements/Current Measurement  PhasorSimulation=off  OutputType=Complex  PSBequivalent=0
  Voltage Measurement : powerlib/Measurements/Voltage Measurement  PhasorSimulation=off  OutputType=Complex  PSBequivalent=0
  prod2 : Product  Inputs=**
  scaling : Subsystem
  unit delay : UnitDelay  SampleTime=1e-4
  in + : PMIOPort  Port=1  Side=Left
  in -- : PMIOPort  Port=2  Side=Left
  out + : PMIOPort  Port=3  Side=Right
  out -- : PMIOPort  Port=4  Side=Right
  m : Outport
  wires:
  prod2/1 -> Bus Creator/4  "Buck Power (W)"
  scaling/1(m) -> unit delay/1
  duty/1 -> scaling/1(D)
  Current Measurement2/1 -> Bus Creator/1  "Buck Inductor Current (A)"
  Current Measurement1/1 -> prod2/1, Bus Creator/2  "Buck Current (A)"
  Voltage Measurement/1 -> prod2/2, Bus Creator/3  "Buck Voltage (V)"
  Bus Creator/1 -> m/1
  unit delay/1 -> Average Voltage Bridge/1
  connections:
  Voltage Measurement/LConn1 -- out +/RConn1 -- Current Measurement1/RConn1
  "1200uF "/LConn1 -- Average Voltage Bridge/RConn1 -- in +/RConn1
  in --/RConn1 -- "1200uF "/RConn1 -- Average Voltage Bridge/RConn2
  402uH/RConn1 -- Average Voltage Bridge/LConn1
  out --/RConn1 -- 1200uF/RConn1 -- Voltage Measurement/LConn2
  Current Measurement1/LConn1 -- 1200uF/LConn1 -- Current Measurement2/RConn1
  402uH/LConn1 -- Current Measurement2/LConn1

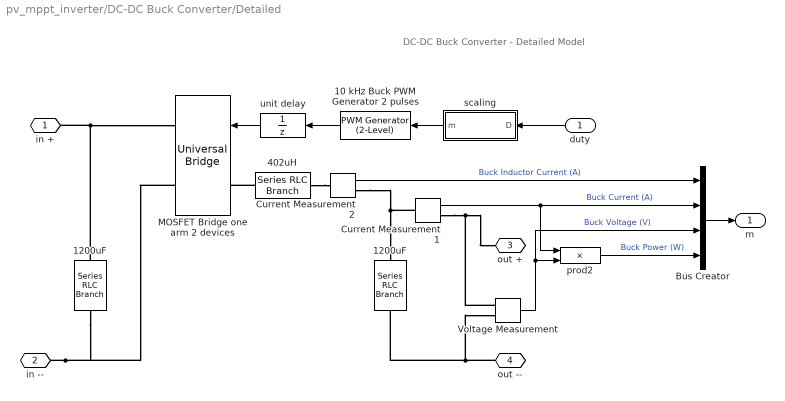
== system pv_mppt_inverter/DC-DC Buck Converter/Detailed ==
  note: DC-DC Buck Converter - Detailed Model
  duty : Inport
  10 kHz Buck PWM Generator 2 pulses : powerlib_meascontrol/Pulse & Signal Generators/PWM Generator (2-Level)  ModulatorType=Single-phase half-bridge (2 pulses)  ModulatorMode=Unsynchronized  nF=27  Fc=1e04  ModulatingSignals=off  m=0.8  Freq=60  Phase=0  Ts=Ts
  1200uF : powerlib/Elements/Series RLC Branch  LConnTagsString=__new0  RConnTagsString=__new0  BranchType=RC  Resistance=0.25  Inductance=30e-6  SetiL0=off  InitialCurrent=0  Capacitance=1200e-6  Setx0=on  InitialVoltage=157  Measurements=None
  "1200uF " : powerlib/Elements/Series RLC Branch  LConnTagsString=__new0  RConnTagsString=__new0  BranchType=RC  Resistance=0.25  Inductance=30e-6  SetiL0=off  InitialCurrent=0  Capacitance=1200e-6  Setx0=on  InitialVoltage=196  Measurements=None
  402uH : powerlib/Elements/Series RLC Branch  LConnTagsString=__new0  RConnTagsString=__new0  BranchType=RL  Resistance=0.1  Inductance=402e-6  SetiL0=off  InitialCurrent=18  Capacitance=1e-6  Setx0=off  InitialVoltage=0  Measurements=None
  Bus Creator : BusCreator
  Current Measurement1 : powerlib/Measurements/Current Measurement  PhasorSimulation=off  OutputType=Complex  PSBequivalent=0
  Current Measurement2 : powerlib/Measurements/Current Measurement  PhasorSimulation=off  OutputType=Complex  PSBequivalent=0
  MOSFET Bridge one arm 2 devices : powerlib/Power Electronics/Universal Bridge  Arms=1  SnubberResistance=1e5  SnubberCapacitance=inf  Device=MOSFET / Diodes  Ron=1e-4  Lon=0  ForwardVoltages="[  0  0  ]"  ForwardVoltage=0  GTOparameters=[ 10e-6 , 20e-6 ]  IGBTparameters=[ 1e-6 , 2e-6 ]  Measurements=None  Measurements_2=None  converterType=Rectifier
  Voltage Measurement : powerlib/Measurements/Voltage Measurement  PhasorSimulation=off  OutputType=Complex  PSBequivalent=0
  prod2 : Product  Inputs=**
  scaling : Subsystem
  unit delay : UnitDelay  SampleTime=Ts
  in + : PMIOPort  Port=1  Side=Left
  in -- : PMIOPort  Port=2  Side=Left
  out + : PMIOPort  Port=3  Side=Right
  out -- : PMIOPort  Port=4  Side=Right
  m : Outport
  wires:
  10 kHz Buck PWM Generator 2 pulses/1 -> unit delay/1
  prod2/1 -> Bus Creator/4  "Buck Power (W)"
  scaling/1(m) -> 10 kHz Buck PWM Generator 2 pulses/1
  duty/1 -> scaling/1(D)
  Current Measurement2/1 -> Bus Creator/1  "Buck Inductor Current (A)"
  Current Measurement1/1 -> prod2/1, Bus Creator/2  "Buck Current (A)"
  Voltage Measurement/1 -> prod2/2, Bus Creator/3  "Buck Voltage (V)"
  Bus Creator/1 -> m/1
  unit delay/1 -> MOSFET Bridge one arm 2 devices/1
  connections:
  Voltage Measurement/LConn1 -- out +/RConn1 -- Current Measurement1/RConn1
  "1200uF "/LConn1 -- MOSFET Bridge one arm 2 devices/RConn1 -- in +/RConn1
  in --/RConn1 -- "1200uF "/RConn1 -- MOSFET Bridge one arm 2 devices/RConn2
  402uH/RConn1 -- MOSFET Bridge one arm 2 devices/LConn1
  out --/RConn1 -- 1200uF/RConn1 -- Voltage Measurement/LConn2
  Current Measurement1/LConn1 -- 1200uF/LConn1 -- Current Measurement2/RConn1
  402uH/LConn1 -- Current Measurement2/LConn1

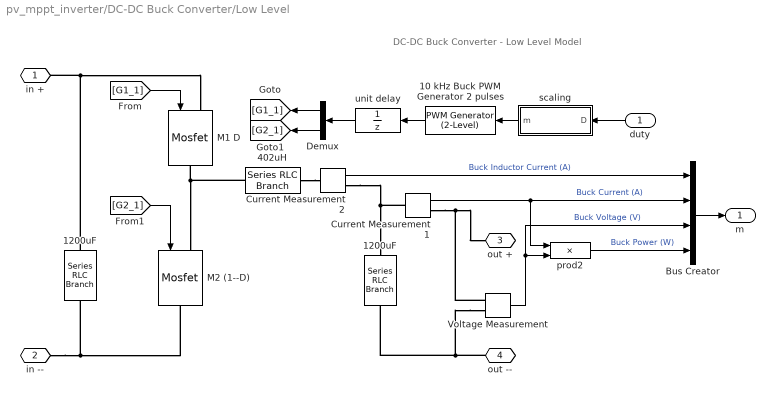
== system pv_mppt_inverter/DC-DC Buck Converter/Low Level ==
  note: DC-DC Buck Converter - Low Level Model
  duty : Inport
  10 kHz Buck PWM Generator 2 pulses : powerlib_meascontrol/Pulse & Signal Generators/PWM Generator (2-Level)  ModulatorType=Single-phase half-bridge (2 pulses)  ModulatorMode=Unsynchronized  nF=27  Fc=1e04  ModulatingSignals=off  m=0.8  Freq=60  Phase=0  Ts=Ts
  1200uF : powerlib/Elements/Series RLC Branch  LConnTagsString=__new0  RConnTagsString=__new0  BranchType=RC  Resistance=0.25  Inductance=30e-6  SetiL0=off  InitialCurrent=0  Capacitance=1200e-6  Setx0=on  InitialVoltage=157  Measurements=None
  "1200uF " : powerlib/Elements/Series RLC Branch  LConnTagsString=__new0  RConnTagsString=__new0  BranchType=RC  Resistance=0.25  Inductance=30e-6  SetiL0=off  InitialCurrent=0  Capacitance=1200e-6  Setx0=on  InitialVoltage=196  Measurements=None
  402uH : powerlib/Elements/Series RLC Branch  LConnTagsString=__new0  RConnTagsString=__new0  BranchType=RL  Resistance=0.1  Inductance=402e-6  SetiL0=off  InitialCurrent=18  Capacitance=1e-6  Setx0=off  InitialVoltage=0  Measurements=None
  Bus Creator : BusCreator
  Current Measurement1 : powerlib/Measurements/Current Measurement  PhasorSimulation=off  OutputType=Complex  PSBequivalent=0
  Current Measurement2 : powerlib/Measurements/Current Measurement  PhasorSimulation=off  OutputType=Complex  PSBequivalent=0
  Demux : Demux  Outputs=2
  M1 D : powerlib/Power Electronics/Mosfet  Ron=0.001  Lon=0  Rd=0.01  Vfd=0.7  IC=0  Rs=1e5  Cs=inf  Measurements=off
  M2 (1--D) : powerlib/Power Electronics/Mosfet  Ron=0.001  Lon=0  Rd=0.01  Vfd=0.7  IC=0  Rs=1e5  Cs=inf  Measurements=off
  Voltage Measurement : powerlib/Measurements/Voltage Measurement  PhasorSimulation=off  OutputType=Complex  PSBequivalent=0
  prod2 : Product  Inputs=**
  scaling : Subsystem
  unit delay : UnitDelay  SampleTime=Ts
  in + : PMIOPort  Port=1  Side=Left
  in -- : PMIOPort  Port=2  Side=Left
  out + : PMIOPort  Port=3  Side=Right
  out -- : PMIOPort  Port=4  Side=Right
  m : Outport
  wires:
  Bus Creator/1 -> m/1
  Voltage Measurement/1 -> Bus Creator/3, prod2/2  "Buck Voltage (V)"
  Current Measurement1/1 -> Bus Creator/2, prod2/1  "Buck Current (A)"
  Current Measurement2/1 -> Bus Creator/1  "Buck Inductor Current (A)"
  duty/1 -> scaling/1(D)
  scaling/1(m) -> 10 kHz Buck PWM Generator 2 pulses/1
  prod2/1 -> Bus Creator/4  "Buck Power (W)"
  [G2_1] -> M2 (1--D)/1
  Demux/1 -> [G1_1]
  Demux/2 -> [G2_1]
  [G1_1] -> M1 D/1
  10 kHz Buck PWM Generator 2 pulses/1 -> unit delay/1
  unit delay/1 -> Demux/1
  connections:
  402uH/LConn1 -- Current Measurement2/LConn1
  Current Measurement2/RConn1 -- 1200uF/LConn1 -- Current Measurement1/LConn1
  Voltage Measurement/LConn2 -- 1200uF/RConn1 -- out --/RConn1
  402uH/RConn1 -- M2 (1--D)/LConn1 -- M1 D/RConn1
  M2 (1--D)/RConn1 -- "1200uF "/RConn1 -- in --/RConn1
  "1200uF "/LConn1 -- in +/RConn1 -- M1 D/LConn1
  Current Measurement1/RConn1 -- out +/RConn1 -- Voltage Measurement/LConn1

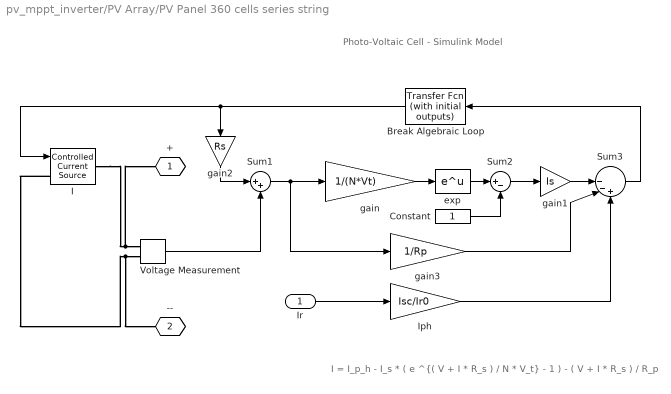
== system pv_mppt_inverter/PV Array/PV Panel 360 cells series string ==
  note: I = I_p_h - I_s * ( e ^{( V + I * R_s ) / N * V_t} - 1 ) - ( V + I * R_s ) / R_p
  note: Photo-Voltaic Cell - Simulink Model
  Ir : Inport
  Break Algebraic Loop : simulink_extras/Additional Linear/Transfer Fcn (with initial outputs)  N=[1]  D="[tau  1]"  Y0=Isc  U0=5.25
  Constant : Constant
  I : powerlib/Electrical Sources/Controlled Current Source  Initialize=on  Source_Type=DC  Amplitude=5  Phase=0  Frequency=0  Measurements=None
  Iph : Gain  Gain=Isc/Ir0
  Sum1 : Sum  Inputs=|++
  Sum2 : Sum  Inputs=|+-
  Sum3 : Sum  Inputs=||--+
  Voltage Measurement : powerlib/Measurements/Voltage Measurement  PhasorSimulation=off  OutputType=Complex  PSBequivalent=0
  exp : Math  SaturateOnIntegerOverflow=on
  gain : Gain  Gain=1/(N*Vt)
  gain1 : Gain  Gain=Is
  gain2 : Gain  Gain=Rs
  gain3 : Gain  Gain=1/Rp
  + : PMIOPort  Tag=PMCPort  Port=1  Side=Right
  -- : PMIOPort  Tag=PMCPort  Port=2  Side=Right
  wires:
  Sum2/1 -> gain1/1
  Constant/1 -> Sum2/2
  exp/1 -> Sum2/1
  Sum1/1 -> gain/1, gain3/1
  gain/1 -> exp/1
  Sum3/1 -> Break Algebraic Loop/1
  Voltage Measurement/1 -> Sum1/2
  Ir/1 -> Iph/1
  Break Algebraic Loop/1 -> gain2/1, I/1
  gain2/1 -> Sum1/1
  gain1/1 -> Sum3/1
  gain3/1 -> Sum3/2
  Iph/1 -> Sum3/3
  connections:
  Voltage Measurement/LConn1 -- +/RConn1 -- I/RConn1
  Voltage Measurement/LConn2 -- --/RConn1 -- I/LConn1

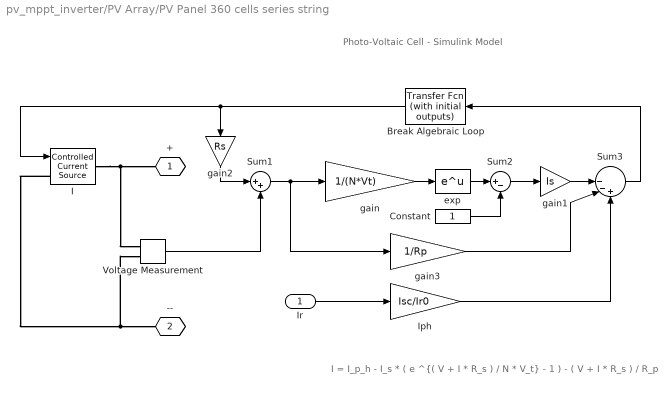
== system pv_mppt_inverter/PV Array/PV Panel 360 cells series string  ==
  note: Photo-Voltaic Cell - Simulink Model
  note: I = I_p_h - I_s * ( e ^{( V + I * R_s ) / N * V_t} - 1 ) - ( V + I * R_s ) / R_p
  Ir : Inport
  Break Algebraic Loop : simulink_extras/Additional Linear/Transfer Fcn (with initial outputs)  N=[1]  D="[tau  1]"  Y0=Isc  U0=5.25
  Constant : Constant
  I : powerlib/Electrical Sources/Controlled Current Source  Initialize=on  Source_Type=DC  Amplitude=5  Phase=0  Frequency=0  Measurements=None
  Iph : Gain  Gain=Isc/Ir0
  Sum1 : Sum  Inputs=|++
  Sum2 : Sum  Inputs=|+-
  Sum3 : Sum  Inputs=||--+
  Voltage Measurement : powerlib/Measurements/Voltage Measurement  PhasorSimulation=off  OutputType=Complex  PSBequivalent=0
  exp : Math  SaturateOnIntegerOverflow=on
  gain : Gain  Gain=1/(N*Vt)
  gain1 : Gain  Gain=Is
  gain2 : Gain  Gain=Rs
  gain3 : Gain  Gain=1/Rp
  + : PMIOPort  Tag=PMCPort  Port=1  Side=Right
  -- : PMIOPort  Tag=PMCPort  Port=2  Side=Right
  wires:
  Iph/1 -> Sum3/3
  gain3/1 -> Sum3/2
  gain1/1 -> Sum3/1
  gain2/1 -> Sum1/1
  Break Algebraic Loop/1 -> I/1, gain2/1
  Ir/1 -> Iph/1
  Voltage Measurement/1 -> Sum1/2
  Sum3/1 -> Break Algebraic Loop/1
  gain/1 -> exp/1
  Sum1/1 -> gain3/1, gain/1
  exp/1 -> Sum2/1
  Constant/1 -> Sum2/2
  Sum2/1 -> gain1/1
  connections:
  I/LConn1 -- --/RConn1 -- Voltage Measurement/LConn2
  I/RConn1 -- +/RConn1 -- Voltage Measurement/LConn1

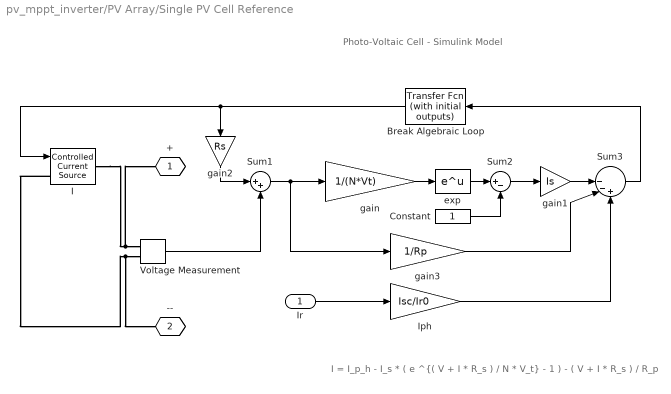
== system pv_mppt_inverter/PV Array/Single PV Cell Reference ==
  note: I = I_p_h - I_s * ( e ^{( V + I * R_s ) / N * V_t} - 1 ) - ( V + I * R_s ) / R_p
  note: Photo-Voltaic Cell - Simulink Model
  Ir : Inport
  Break Algebraic Loop : simulink_extras/Additional Linear/Transfer Fcn (with initial outputs)  N=[1]  D="[tau  1]"  Y0=Isc  U0=0
  Constant : Constant
  I : powerlib/Electrical Sources/Controlled Current Source  Initialize=on  Source_Type=DC  Amplitude=5  Phase=0  Frequency=0  Measurements=None
  Iph : Gain  Gain=Isc/Ir0
  Sum1 : Sum  Inputs=|++
  Sum2 : Sum  Inputs=|+-
  Sum3 : Sum  Inputs=||--+
  Voltage Measurement : powerlib/Measurements/Voltage Measurement  PhasorSimulation=off  OutputType=Complex  PSBequivalent=0
  exp : Math  SaturateOnIntegerOverflow=on
  gain : Gain  Gain=1/(N*Vt)
  gain1 : Gain  Gain=Is
  gain2 : Gain  Gain=Rs
  gain3 : Gain  Gain=1/Rp
  + : PMIOPort  Tag=PMCPort  Port=1  Side=Right
  -- : PMIOPort  Tag=PMCPort  Port=2  Side=Right
  wires:
  Sum2/1 -> gain1/1
  Constant/1 -> Sum2/2
  exp/1 -> Sum2/1
  Sum1/1 -> gain/1, gain3/1
  gain/1 -> exp/1
  Sum3/1 -> Break Algebraic Loop/1
  Voltage Measurement/1 -> Sum1/2
  Ir/1 -> Iph/1
  Break Algebraic Loop/1 -> gain2/1, I/1
  gain2/1 -> Sum1/1
  gain1/1 -> Sum3/1
  gain3/1 -> Sum3/2
  Iph/1 -> Sum3/3
  connections:
  Voltage Measurement/LConn1 -- +/RConn1 -- I/RConn1
  Voltage Measurement/LConn2 -- --/RConn1 -- I/LConn1

== system pv_mppt_inverter/DC-DC Buck Converter/AVG Voltage/scaling ==
  note: Shifting from ]0 to 1[ to a ]-1 to 1[ scale
  D : Inport
  Bias : Bias  Bias=-0.5
  Gain : Gain  Gain=2
  Saturation : Saturate  UpperLimit=1  LowerLimit=-1
  m : Outport
  wires:
  Bias/1 -> Gain/1
  D/1 -> Bias/1
  Gain/1 -> Saturation/1
  Saturation/1 -> m/1

== system pv_mppt_inverter/DC-DC Buck Converter/Detailed/scaling ==
  note: Shifting from ]0 to 1[ to a ]-1 to 1[ scale
  D : Inport
  Bias : Bias  Bias=-0.5
  Gain : Gain  Gain=2
  Saturation : Saturate  UpperLimit=1  LowerLimit=-1
  m : Outport
  wires:
  Bias/1 -> Gain/1
  D/1 -> Bias/1
  Gain/1 -> Saturation/1
  Saturation/1 -> m/1

== system pv_mppt_inverter/DC-DC Buck Converter/Low Level/scaling ==
  note: Shifting from ]0 to 1[ to a ]-1 to 1[ scale
  D : Inport
  Bias : Bias  Bias=-0.5
  Gain : Gain  Gain=2
  Saturation : Saturate  UpperLimit=1  LowerLimit=-1
  m : Outport
  wires:
  Saturation/1 -> m/1
  Gain/1 -> Saturation/1
  D/1 -> Bias/1
  Bias/1 -> Gain/1
